simulink model "sistemaLinearOrdem3"  (R2018a)
settings: Solver=VariableStepAuto  StartTime=0.0  StopTime=20  MaxStep=.1  RelTol=1e-3
model workspace (MAT data in the model file):
  p = [0.1 0.122448979592 0.144897959184 0.167346938776 0.189795918367 0.212244897959 0.234693877551 0.257142857143 0.279591836735 0.302040816327 0.324489795918 0.34693877551 0.369387755102 0.391836734694 0.414285714286 0.436734693878 0.459183673469 0.481632653061 0.504081632653 0.526530612245 0.548979591837 0.571428571429 0.59387755102 0.616326530612 0.638775510204 0.661224489796 0.683673469388 0.70612244898 0.728571428571 0.751020408163 0.773469387755 0.795918367347 0.818367346939 0.840816326531 0.863265306122 0.885714285714 0.908163265306 0.930612244898 0.95306122449 0.975510204082 0.997959183673 1.02040816327 1.04285714286 1.06530612245 1.08775510204 1.11020408163 1.13265306122 1.15510204082 1.17755102041 1.2]
settings Model: Creator=gnsoares  LastModifiedBy=gnsoares

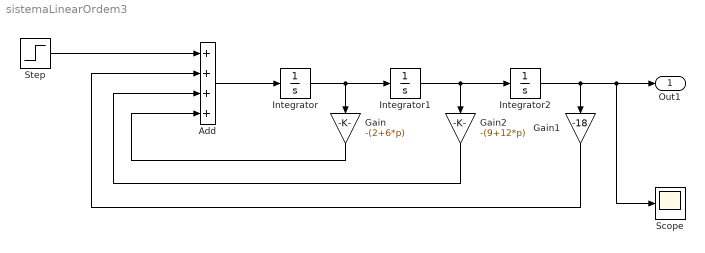
== system sistemaLinearOrdem3 ==
  Add : Sum  Inputs=++++
  Gain : Gain  Gain=-(2+6*p)
  Gain1 : Gain  Gain=-18
  Gain2 : Gain  Gain=-(9+12*p)
  Integrator : Integrator
  Integrator1 : Integrator
  Integrator2 : Integrator
  Scope : Scope
  Step : Step  Time=0  After=18  SampleTime=0
  Out1 : Outport
  wires:
  Step/1 -> Add/1
  Add/1 -> Integrator/1
  Integrator/1 -> Integrator1/1, Gain/1
  Integrator1/1 -> Integrator2/1, Gain2/1
  Integrator2/1 -> Scope/1, Out1/1, Gain1/1
  Gain/1 -> Add/4
  Gain2/1 -> Add/3
  Gain1/1 -> Add/2
